simulink model "Controller_Exp"  (R2016a)
settings: Solver=ode4  StartTime=0.0  StopTime=Inf  FixedStep=Ts  RelTol=1e-3
undefined symbols (not defined in the file or in its folder): A_lpf_velocity, B1_lpf_velocity, B2_lpf_velocity, Calibration, commanded_u, GearOffsets, IMUTorsoOffsets, MedullaCommand, ResetDAQ, sample_time, TorsoCOMOffsets, Ts
libraries: xpcethercatlib x188, simulink x37, slrtlib x11, ControllerLibrary x2, dspswit3 x1
(part 2 of 4)

== system Controller_Exp/DAQ/DAQ_sub/Subsystem/EncoderFilters/Filter ==
  note: Look at 10 Samples to determine if there are any spikes in the data.
      | If so, take the median of the 10 samples.
  q : Inport
  Delay : Delay  DelayLength=1
  Delay1 : Delay
  Delay2 : Delay  DelayLength=3
  Delay3 : Delay  DelayLength=4
  Delay4 : Delay  DelayLength=5
  Delay5 : Delay  DelayLength=6
  Delay6 : Delay  DelayLength=7
  Delay7 : Delay  DelayLength=8
  Delay8 : Delay  DelayLength=9
  Median Filter : MATLAB Function  TreatAsAtomicUnit=on
  Vector Concatenate : Concatenate  NumInputs=9  Mode=Multidimensional array  ConcatenateDimension=2
  Velocity Filter : Subsystem
  q_clean : Outport
  dq_clean : Outport  Port=2
  dq_clean_original : Outport  Port=3
  wires:
  Vector Concatenate/1 -> Median Filter/2(q_past)
  Delay/1 -> Vector Concatenate/1
  Delay1/1 -> Vector Concatenate/2
  Delay2/1 -> Vector Concatenate/3
  Delay3/1 -> Vector Concatenate/4
  Delay4/1 -> Vector Concatenate/5
  Delay5/1 -> Vector Concatenate/6
  Delay6/1 -> Vector Concatenate/7
  Delay7/1 -> Vector Concatenate/8
  Delay8/1 -> Vector Concatenate/9
  q/1 -> Delay8/1, Delay7/1, Delay6/1, Delay5/1, Delay4/1, Delay3/1, Delay2/1, Delay1/1, Delay/1, Median Filter/1(q)
  Velocity Filter/2(dq_original) -> dq_clean_original/1
  Velocity Filter/1(dq_out) -> dq_clean/1
  Median Filter/1(q_out) -> Velocity Filter/1(q), q_clean/1

== system Controller_Exp/DAQ/DAQ_sub/Subsystem/EncoderFilters1/CheckAndFilterEncoder ==
  q_daq : Inport
  Logic Filter : MATLAB Function  TreatAsAtomicUnit=on
  Unit Delay1 : UnitDelay  SampleTime=-1
  Unit Delay2 : UnitDelay  SampleTime=-1
  Velocity Filter : Subsystem
  q_clean : Outport
  dq_clean : Outport  Port=2
  dq_clean_origin : Outport  Port=3
  wires:
  Velocity Filter/2(Out2) -> dq_clean_origin/1
  Velocity Filter/1(Out1) -> dq_clean/1
  q_daq/1 -> Unit Delay2/1, Logic Filter/1(q)
  Logic Filter/1(q_out) -> q_clean/1, Velocity Filter/1(In1)
  Logic Filter/2(q_good) -> Unit Delay1/1
  Unit Delay1/1 -> Logic Filter/3(q_good_prev)
  Unit Delay2/1 -> Logic Filter/2(q_prev)

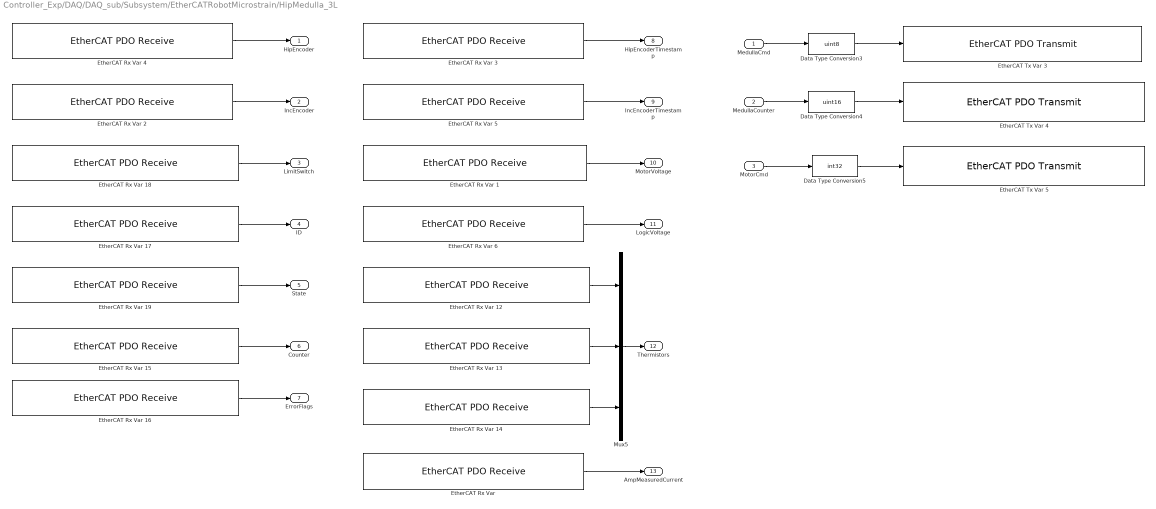
== system Controller_Exp/DAQ/DAQ_sub/Subsystem/EtherCATRobotMicrostrain/HipMedulla_3L ==
  MedullaCmd : Inport
  MedullaCounter : Inport  Port=2
  MotorCmd : Inport  Port=3
  Data Type Conversion3 : DataTypeConversion  OutDataTypeStr=uint8  RndMeth=Simplest
  Data Type Conversion4 : DataTypeConversion  OutDataTypeStr=uint16  RndMeth=Simplest
  Data Type Conversion5 : DataTypeConversion  OutDataTypeStr=int32  RndMeth=Simplest
  "EtherCAT Rx Var " : xpcethercatlib/EtherCAT PDO Receive  Priority=2  sig_name=Box 1 (ATRIAS 2.1 Hip (Medulla 1.5)).Measured Current.Amp Measured Current  sig_offset=760  sig_type=int16  type_size=16  sig_dim=1  device_id=3  sample_time=0.001000
  EtherCAT Rx Var 1 : xpcethercatlib/EtherCAT PDO Receive  Priority=2  sig_name=Box 1 (ATRIAS 2.1 Hip (Medulla 1.5)).Power.Motor Voltage  sig_offset=680  sig_type=uint16  type_size=16  sig_dim=1  device_id=3  sample_time=0.001000
  EtherCAT Rx Var 12 : xpcethercatlib/EtherCAT PDO Receive  Priority=2  sig_name=Box 1 (ATRIAS 2.1 Hip (Medulla 1.5)).Thermistors.Thermistor 0  sig_offset=712  sig_type=uint16  type_size=16  sig_dim=1  device_id=3  sample_time=0.001000
  EtherCAT Rx Var 13 : xpcethercatlib/EtherCAT PDO Receive  Priority=2  sig_name=Box 1 (ATRIAS 2.1 Hip (Medulla 1.5)).Thermistors.Thermistor 1  sig_offset=728  sig_type=uint16  type_size=16  sig_dim=1  device_id=3  sample_time=0.001000
  EtherCAT Rx Var 14 : xpcethercatlib/EtherCAT PDO Receive  Priority=2  sig_name=Box 1 (ATRIAS 2.1 Hip (Medulla 1.5)).Thermistors.Thermistor 2  sig_offset=744  sig_type=uint16  type_size=16  sig_dim=1  device_id=3  sample_time=0.001000
  EtherCAT Rx Var 15 : xpcethercatlib/EtherCAT PDO Receive  Priority=2  sig_name=Box 1 (ATRIAS 2.1 Hip (Medulla 1.5)).uController Status.Counter  sig_offset=608  sig_type=uint8  type_size=8  sig_dim=1  device_id=3  sample_time=0.001000
  EtherCAT Rx Var 16 : xpcethercatlib/EtherCAT PDO Receive  Priority=2  sig_name=Box 1 (ATRIAS 2.1 Hip (Medulla 1.5)).uController Status.Error Flags  sig_offset=616  sig_type=uint8  type_size=8  sig_dim=1  device_id=3  sample_time=0.001000
  EtherCAT Rx Var 17 : xpcethercatlib/EtherCAT PDO Receive  Priority=2  sig_name=Box 1 (ATRIAS 2.1 Hip (Medulla 1.5)).uController Status.ID  sig_offset=592  sig_type=uint8  type_size=8  sig_dim=1  device_id=3  sample_time=0.001000
  EtherCAT Rx Var 18 : xpcethercatlib/EtherCAT PDO Receive  Priority=2  sig_name=Box 1 (ATRIAS 2.1 Hip (Medulla 1.5)).uController Status.Limit Switch  sig_offset=624  sig_type=uint8  type_size=8  sig_dim=1  device_id=3  sample_time=0.001000
  EtherCAT Rx Var 19 : xpcethercatlib/EtherCAT PDO Receive  Priority=2  sig_name=Box 1 (ATRIAS 2.1 Hip (Medulla 1.5)).uController Status.State  sig_offset=600  sig_type=uint8  type_size=8  sig_dim=1  device_id=3  sample_time=0.001000
  EtherCAT Rx Var 2 : xpcethercatlib/EtherCAT PDO Receive  Priority=2  sig_name=Box 1 (ATRIAS 2.1 Hip (Medulla 1.5)).Incremental Encoder.Incremental Encoder  sig_offset=776  sig_type=uint16  type_size=16  sig_dim=1  device_id=3  sample_time=0.001000
  EtherCAT Rx Var 3 : xpcethercatlib/EtherCAT PDO Receive  Priority=2  sig_name=Box 1 (ATRIAS 2.1 Hip (Medulla 1.5)).Hip Encoder.Timestamp  sig_offset=664  sig_type=uint16  type_size=16  sig_dim=1  device_id=3  sample_time=0.001000
  EtherCAT Rx Var 4 : xpcethercatlib/EtherCAT PDO Receive  Priority=2  sig_name=Box 1 (ATRIAS 2.1 Hip (Medulla 1.5)).Hip Encoder.Encoder  sig_offset=632  sig_type=uint32  type_size=32  sig_dim=1  device_id=3  sample_time=0.001000
  EtherCAT Rx Var 5 : xpcethercatlib/EtherCAT PDO Receive  Priority=2  sig_name=Box 1 (ATRIAS 2.1 Hip (Medulla 1.5)).Incremental Encoder.Incremental Encoder Timestamp  sig_offset=792  sig_type=uint16  type_size=16  sig_dim=1  device_id=3  sample_time=0.001000
  EtherCAT Rx Var 6 : xpcethercatlib/EtherCAT PDO Receive  Priority=2  sig_name=Box 1 (ATRIAS 2.1 Hip (Medulla 1.5)).Power.Logic Voltage  sig_offset=696  sig_type=uint16  type_size=16  sig_dim=1  device_id=3  sample_time=0.001000
  EtherCAT Tx Var 3 : xpcethercatlib/EtherCAT PDO Transmit   Priority=3  sig_name=Box 1 (ATRIAS 2.1 Hip (Medulla 1.5)).uControllerInput.Command  sig_offset=592  sig_type=uint8  type_size=8  sig_dim=1  device_id=3  sample_time=0.001000
  EtherCAT Tx Var 4 : xpcethercatlib/EtherCAT PDO Transmit   Priority=3  sig_name=Box 1 (ATRIAS 2.1 Hip (Medulla 1.5)).uControllerInput.Counter  sig_offset=600  sig_type=uint16  type_size=16  sig_dim=1  device_id=3  sample_time=0.001000
  EtherCAT Tx Var 5 : xpcethercatlib/EtherCAT PDO Transmit   Priority=3  sig_name=Box 1 (ATRIAS 2.1 Hip (Medulla 1.5)).uControllerInput.Motor Current  sig_offset=616  sig_type=int32  type_size=32  sig_dim=1  device_id=3  sample_time=0.001000
  Mux5 : Mux  Inputs=3
  HipEncoder : Outport
  IncEncoder : Outport  Port=2
  LimitSwitch : Outport  Port=3
  ID : Outport  Port=4
  State : Outport  Port=5
  Counter : Outport  Port=6
  ErrorFlags : Outport  Port=7
  HipEncoderTimestamp : Outport  Port=8
  IncEncoderTimestamp : Outport  Port=9
  MotorVoltage : Outport  Port=10
  LogicVoltage : Outport  Port=11
  Thermistors : Outport  Port=12
  AmpMeasuredCurrent : Outport  Port=13
  wires:
  Mux5/1 -> Thermistors/1
  "EtherCAT Rx Var "/1 -> AmpMeasuredCurrent/1
  EtherCAT Rx Var 14/1 -> Mux5/3
  EtherCAT Rx Var 13/1 -> Mux5/2
  EtherCAT Rx Var 12/1 -> Mux5/1
  EtherCAT Rx Var 1/1 -> MotorVoltage/1
  EtherCAT Rx Var 6/1 -> LogicVoltage/1
  EtherCAT Rx Var 16/1 -> ErrorFlags/1
  EtherCAT Rx Var 19/1 -> State/1
  EtherCAT Rx Var 18/1 -> LimitSwitch/1
  EtherCAT Rx Var 17/1 -> ID/1
  EtherCAT Rx Var 15/1 -> Counter/1
  EtherCAT Rx Var 2/1 -> IncEncoder/1
  EtherCAT Rx Var 3/1 -> HipEncoderTimestamp/1
  EtherCAT Rx Var 4/1 -> HipEncoder/1
  EtherCAT Rx Var 5/1 -> IncEncoderTimestamp/1
  MotorCmd/1 -> Data Type Conversion5/1
  MedullaCounter/1 -> Data Type Conversion4/1
  MedullaCmd/1 -> Data Type Conversion3/1
  Data Type Conversion5/1 -> EtherCAT Tx Var 5/1
  Data Type Conversion4/1 -> EtherCAT Tx Var 4/1
  Data Type Conversion3/1 -> EtherCAT Tx Var 3/1

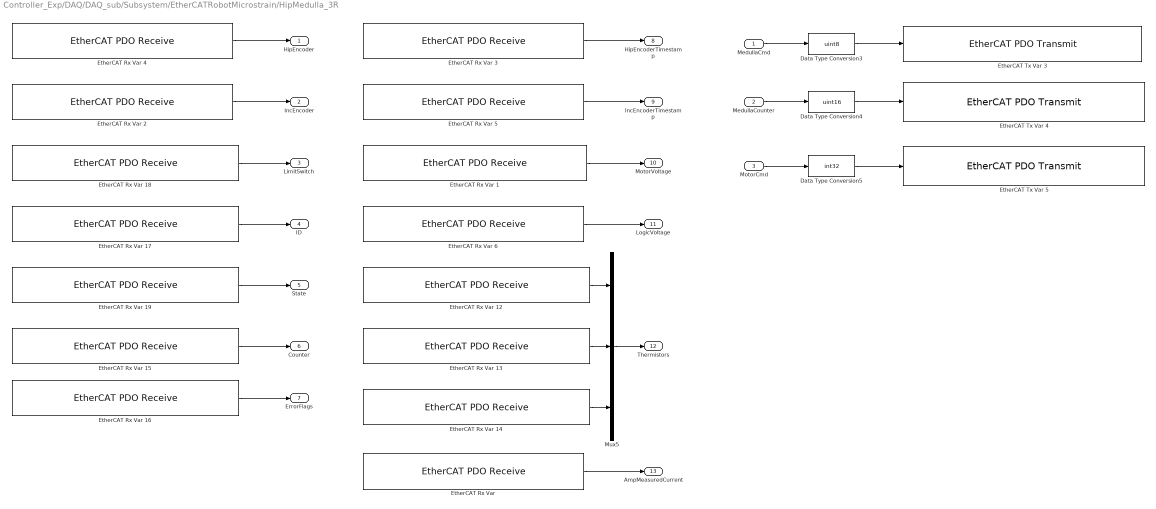
== system Controller_Exp/DAQ/DAQ_sub/Subsystem/EtherCATRobotMicrostrain/HipMedulla_3R ==
  MedullaCmd : Inport
  MedullaCounter : Inport  Port=2
  MotorCmd : Inport  Port=3
  Data Type Conversion3 : DataTypeConversion  OutDataTypeStr=uint8  RndMeth=Simplest
  Data Type Conversion4 : DataTypeConversion  OutDataTypeStr=uint16  RndMeth=Simplest
  Data Type Conversion5 : DataTypeConversion  OutDataTypeStr=int32  RndMeth=Simplest
  "EtherCAT Rx Var " : xpcethercatlib/EtherCAT PDO Receive  Priority=2  sig_name=Box 11 (ATRIAS 2.1 Hip (Medulla 1.5)).Measured Current.Amp Measured Current  sig_offset=2768  sig_type=int16  type_size=16  sig_dim=1  device_id=3  sample_time=0.001000
  EtherCAT Rx Var 1 : xpcethercatlib/EtherCAT PDO Receive  Priority=2  sig_name=Box 11 (ATRIAS 2.1 Hip (Medulla 1.5)).Power.Motor Voltage  sig_offset=2688  sig_type=uint16  type_size=16  sig_dim=1  device_id=3  sample_time=0.001000
  EtherCAT Rx Var 12 : xpcethercatlib/EtherCAT PDO Receive  Priority=2  sig_name=Box 11 (ATRIAS 2.1 Hip (Medulla 1.5)).Thermistors.Thermistor 0  sig_offset=2720  sig_type=uint16  type_size=16  sig_dim=1  device_id=3  sample_time=0.001000
  EtherCAT Rx Var 13 : xpcethercatlib/EtherCAT PDO Receive  Priority=2  sig_name=Box 11 (ATRIAS 2.1 Hip (Medulla 1.5)).Thermistors.Thermistor 1  sig_offset=2736  sig_type=uint16  type_size=16  sig_dim=1  device_id=3  sample_time=0.001000
  EtherCAT Rx Var 14 : xpcethercatlib/EtherCAT PDO Receive  Priority=2  sig_name=Box 11 (ATRIAS 2.1 Hip (Medulla 1.5)).Thermistors.Thermistor 2  sig_offset=2752  sig_type=uint16  type_size=16  sig_dim=1  device_id=3  sample_time=0.001000
  EtherCAT Rx Var 15 : xpcethercatlib/EtherCAT PDO Receive  Priority=2  sig_name=Box 11 (ATRIAS 2.1 Hip (Medulla 1.5)).uController Status.Counter  sig_offset=2616  sig_type=uint8  type_size=8  sig_dim=1  device_id=3  sample_time=0.001000
  EtherCAT Rx Var 16 : xpcethercatlib/EtherCAT PDO Receive  Priority=2  sig_name=Box 11 (ATRIAS 2.1 Hip (Medulla 1.5)).uController Status.Error Flags  sig_offset=2624  sig_type=uint8  type_size=8  sig_dim=1  device_id=3  sample_time=0.001000
  EtherCAT Rx Var 17 : xpcethercatlib/EtherCAT PDO Receive  Priority=2  sig_name=Box 11 (ATRIAS 2.1 Hip (Medulla 1.5)).uController Status.ID  sig_offset=2600  sig_type=uint8  type_size=8  sig_dim=1  device_id=3  sample_time=0.001000
  EtherCAT Rx Var 18 : xpcethercatlib/EtherCAT PDO Receive  Priority=2  sig_name=Box 11 (ATRIAS 2.1 Hip (Medulla 1.5)).uController Status.Limit Switch  sig_offset=2632  sig_type=uint8  type_size=8  sig_dim=1  device_id=3  sample_time=0.001000
  EtherCAT Rx Var 19 : xpcethercatlib/EtherCAT PDO Receive  Priority=2  sig_name=Box 11 (ATRIAS 2.1 Hip (Medulla 1.5)).uController Status.State  sig_offset=2608  sig_type=uint8  type_size=8  sig_dim=1  device_id=3  sample_time=0.001000
  EtherCAT Rx Var 2 : xpcethercatlib/EtherCAT PDO Receive  Priority=2  sig_name=Box 11 (ATRIAS 2.1 Hip (Medulla 1.5)).Incremental Encoder.Incremental Encoder  sig_offset=2784  sig_type=uint16  type_size=16  sig_dim=1  device_id=3  sample_time=0.001000
  EtherCAT Rx Var 3 : xpcethercatlib/EtherCAT PDO Receive  Priority=2  sig_name=Box 11 (ATRIAS 2.1 Hip (Medulla 1.5)).Hip Encoder.Timestamp  sig_offset=2672  sig_type=uint16  type_size=16  sig_dim=1  device_id=3  sample_time=0.001000
  EtherCAT Rx Var 4 : xpcethercatlib/EtherCAT PDO Receive  Priority=2  sig_name=Box 11 (ATRIAS 2.1 Hip (Medulla 1.5)).Hip Encoder.Encoder  sig_offset=2640  sig_type=uint32  type_size=32  sig_dim=1  device_id=3  sample_time=0.001000
  EtherCAT Rx Var 5 : xpcethercatlib/EtherCAT PDO Receive  Priority=2  sig_name=Box 11 (ATRIAS 2.1 Hip (Medulla 1.5)).Incremental Encoder.Incremental Encoder Timestamp  sig_offset=2800  sig_type=uint16  type_size=16  sig_dim=1  device_id=3  sample_time=0.001000
  EtherCAT Rx Var 6 : xpcethercatlib/EtherCAT PDO Receive  Priority=2  sig_name=Box 11 (ATRIAS 2.1 Hip (Medulla 1.5)).Power.Logic Voltage  sig_offset=2704  sig_type=uint16  type_size=16  sig_dim=1  device_id=3  sample_time=0.001000
  EtherCAT Tx Var 3 : xpcethercatlib/EtherCAT PDO Transmit   Priority=3  sig_name=Box 11 (ATRIAS 2.1 Hip (Medulla 1.5)).uControllerInput.Command  sig_offset=2600  sig_type=uint8  type_size=8  sig_dim=1  device_id=3  sample_time=0.001000
  EtherCAT Tx Var 4 : xpcethercatlib/EtherCAT PDO Transmit   Priority=3  sig_name=Box 11 (ATRIAS 2.1 Hip (Medulla 1.5)).uControllerInput.Counter  sig_offset=2608  sig_type=uint16  type_size=16  sig_dim=1  device_id=3  sample_time=0.001000
  EtherCAT Tx Var 5 : xpcethercatlib/EtherCAT PDO Transmit   Priority=3  sig_name=Box 11 (ATRIAS 2.1 Hip (Medulla 1.5)).uControllerInput.Motor Current  sig_offset=2624  sig_type=int32  type_size=32  sig_dim=1  device_id=3  sample_time=0.001000
  Mux5 : Mux  Inputs=3
  HipEncoder : Outport
  IncEncoder : Outport  Port=2
  LimitSwitch : Outport  Port=3
  ID : Outport  Port=4
  State : Outport  Port=5
  Counter : Outport  Port=6
  ErrorFlags : Outport  Port=7
  HipEncoderTimestamp : Outport  Port=8
  IncEncoderTimestamp : Outport  Port=9
  MotorVoltage : Outport  Port=10
  LogicVoltage : Outport  Port=11
  Thermistors : Outport  Port=12
  AmpMeasuredCurrent : Outport  Port=13
  wires:
  Mux5/1 -> Thermistors/1
  "EtherCAT Rx Var "/1 -> AmpMeasuredCurrent/1
  EtherCAT Rx Var 14/1 -> Mux5/3
  EtherCAT Rx Var 13/1 -> Mux5/2
  EtherCAT Rx Var 12/1 -> Mux5/1
  EtherCAT Rx Var 1/1 -> MotorVoltage/1
  EtherCAT Rx Var 6/1 -> LogicVoltage/1
  EtherCAT Rx Var 16/1 -> ErrorFlags/1
  EtherCAT Rx Var 19/1 -> State/1
  EtherCAT Rx Var 18/1 -> LimitSwitch/1
  EtherCAT Rx Var 17/1 -> ID/1
  EtherCAT Rx Var 15/1 -> Counter/1
  EtherCAT Rx Var 2/1 -> IncEncoder/1
  EtherCAT Rx Var 3/1 -> HipEncoderTimestamp/1
  EtherCAT Rx Var 4/1 -> HipEncoder/1
  EtherCAT Rx Var 5/1 -> IncEncoderTimestamp/1
  MotorCmd/1 -> Data Type Conversion5/1
  MedullaCounter/1 -> Data Type Conversion4/1
  MedullaCmd/1 -> Data Type Conversion3/1
  Data Type Conversion5/1 -> EtherCAT Tx Var 5/1
  Data Type Conversion4/1 -> EtherCAT Tx Var 4/1
  Data Type Conversion3/1 -> EtherCAT Tx Var 3/1

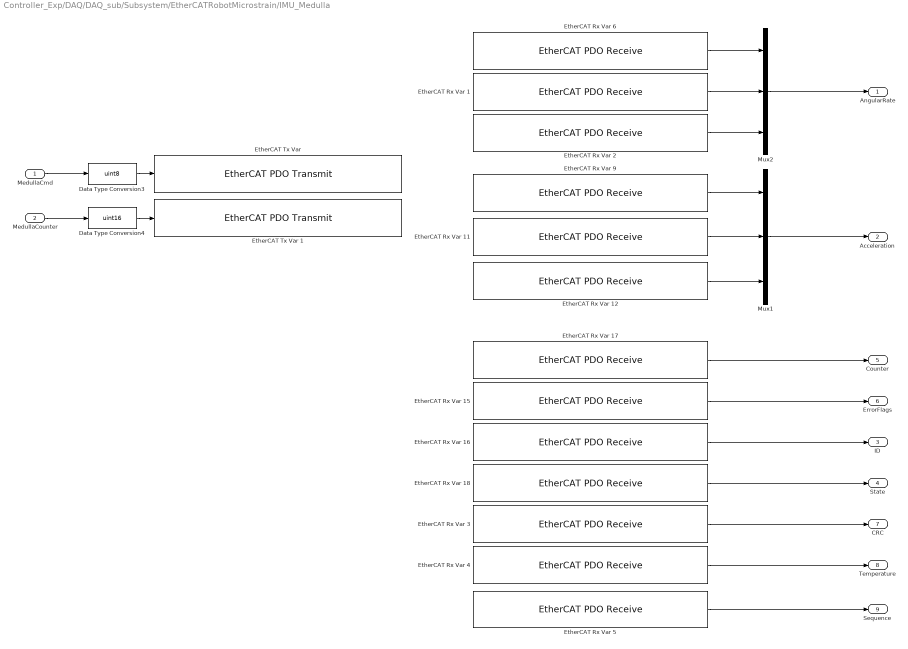
== system Controller_Exp/DAQ/DAQ_sub/Subsystem/EtherCATRobotMicrostrain/IMU_Medulla ==
  MedullaCmd : Inport
  MedullaCounter : Inport  Port=2
  Data Type Conversion3 : DataTypeConversion  OutDataTypeStr=uint8  RndMeth=Simplest
  Data Type Conversion4 : DataTypeConversion  OutDataTypeStr=uint16  RndMeth=Simplest
  EtherCAT Rx Var 1 : xpcethercatlib/EtherCAT PDO Receive  Priority=2  sig_name=Box 4 (ATRIAS 2.1 IMU (Medulla 1.5)).Rotation.Y  sig_offset=872  sig_type=single  type_size=32  sig_dim=1  device_id=3  sample_time=0.001000
  EtherCAT Rx Var 11 : xpcethercatlib/EtherCAT PDO Receive  Priority=2  sig_name=Box 4 (ATRIAS 2.1 IMU (Medulla 1.5)).Acceleration.Y  sig_offset=968  sig_type=single  type_size=32  sig_dim=1  device_id=3  sample_time=0.001000
  EtherCAT Rx Var 12 : xpcethercatlib/EtherCAT PDO Receive  Priority=2  sig_name=Box 4 (ATRIAS 2.1 IMU (Medulla 1.5)).Acceleration.Z  sig_offset=1000  sig_type=single  type_size=32  sig_dim=1  device_id=3  sample_time=0.001000
  EtherCAT Rx Var 15 : xpcethercatlib/EtherCAT PDO Receive  Priority=2  sig_name=Box 4 (ATRIAS 2.1 IMU (Medulla 1.5)).uController Status.Error Flags  sig_offset=832  sig_type=uint8  type_size=8  sig_dim=1  device_id=3  sample_time=0.001000
  EtherCAT Rx Var 16 : xpcethercatlib/EtherCAT PDO Receive  Priority=2  sig_name=Box 4 (ATRIAS 2.1 IMU (Medulla 1.5)).uController Status.ID  sig_offset=808  sig_type=uint8  type_size=8  sig_dim=1  device_id=3  sample_time=0.001000
  EtherCAT Rx Var 17 : xpcethercatlib/EtherCAT PDO Receive  Priority=2  sig_name=Box 4 (ATRIAS 2.1 IMU (Medulla 1.5)).uController Status.Counter  sig_offset=824  sig_type=uint8  type_size=8  sig_dim=1  device_id=3  sample_time=0.001000
  EtherCAT Rx Var 18 : xpcethercatlib/EtherCAT PDO Receive  Priority=2  sig_name=Box 4 (ATRIAS 2.1 IMU (Medulla 1.5)).Status.Status  sig_offset=1032  sig_type=uint8  type_size=8  sig_dim=1  device_id=3  sample_time=0.001000
  EtherCAT Rx Var 2 : xpcethercatlib/EtherCAT PDO Receive  Priority=2  sig_name=Box 4 (ATRIAS 2.1 IMU (Medulla 1.5)).Rotation.Z  sig_offset=904  sig_type=single  type_size=32  sig_dim=1  device_id=3  sample_time=0.001000
  EtherCAT Rx Var 3 : xpcethercatlib/EtherCAT PDO Receive  Priority=2  sig_name=Box 4 (ATRIAS 2.1 IMU (Medulla 1.5)).Status.Status  sig_offset=1032  sig_type=uint8  type_size=8  sig_dim=1  device_id=3  sample_time=0.001000
  EtherCAT Rx Var 4 : xpcethercatlib/EtherCAT PDO Receive  Priority=2  sig_name=Box 4 (ATRIAS 2.1 IMU (Medulla 1.5)).Status.Temperature  sig_offset=1048  sig_type=int16  type_size=16  sig_dim=1  device_id=3  sample_time=0.001000
  EtherCAT Rx Var 5 : xpcethercatlib/EtherCAT PDO Receive  Priority=2  sig_name=Box 4 (ATRIAS 2.1 IMU (Medulla 1.5)).Status.Sequence  sig_offset=1040  sig_type=uint8  type_size=8  sig_dim=1  device_id=3  sample_time=0.001000
  EtherCAT Rx Var 6 : xpcethercatlib/EtherCAT PDO Receive  Priority=2  sig_name=Box 4 (ATRIAS 2.1 IMU (Medulla 1.5)).Rotation.X  sig_offset=840  sig_type=single  type_size=32  sig_dim=1  device_id=3  sample_time=0.001000
  EtherCAT Rx Var 9 : xpcethercatlib/EtherCAT PDO Receive  Priority=2  sig_name=Box 4 (ATRIAS 2.1 IMU (Medulla 1.5)).Acceleration.X  sig_offset=936  sig_type=single  type_size=32  sig_dim=1  device_id=3  sample_time=0.001000
  "EtherCAT Tx Var " : xpcethercatlib/EtherCAT PDO Transmit   Priority=3  sig_name=Box 4 (ATRIAS 2.1 IMU (Medulla 1.5)).uControllerInput.Command  sig_offset=808  sig_type=uint8  type_size=8  sig_dim=1  device_id=3  sample_time=0.001000
  EtherCAT Tx Var 1 : xpcethercatlib/EtherCAT PDO Transmit   Priority=3  sig_name=Box 4 (ATRIAS 2.1 IMU (Medulla 1.5)).uControllerInput.Counter  sig_offset=816  sig_type=uint16  type_size=16  sig_dim=1  device_id=3  sample_time=0.001000
  Mux1 : Mux  Inputs=3
  Mux2 : Mux  Inputs=3
  AngularRate : Outport
  Acceleration : Outport  Port=2
  ID : Outport  Port=3
  State : Outport  Port=4
  Counter : Outport  Port=5
  ErrorFlags : Outport  Port=6
  CRC : Outport  Port=7
  Temperature : Outport  Port=8
  Sequence : Outport  Port=9
  wires:
  EtherCAT Rx Var 6/1 -> Mux2/1
  EtherCAT Rx Var 2/1 -> Mux2/3
  EtherCAT Rx Var 1/1 -> Mux2/2
  Mux2/1 -> AngularRate/1
  EtherCAT Rx Var 9/1 -> Mux1/1
  EtherCAT Rx Var 11/1 -> Mux1/2
  EtherCAT Rx Var 12/1 -> Mux1/3
  EtherCAT Rx Var 18/1 -> State/1
  EtherCAT Rx Var 16/1 -> ID/1
  EtherCAT Rx Var 15/1 -> ErrorFlags/1
  EtherCAT Rx Var 17/1 -> Counter/1
  MedullaCounter/1 -> Data Type Conversion4/1
  MedullaCmd/1 -> Data Type Conversion3/1
  Data Type Conversion4/1 -> EtherCAT Tx Var 1/1
  Data Type Conversion3/1 -> "EtherCAT Tx Var "/1
  Mux1/1 -> Acceleration/1
  EtherCAT Rx Var 3/1 -> CRC/1
  EtherCAT Rx Var 4/1 -> Temperature/1
  EtherCAT Rx Var 5/1 -> Sequence/1

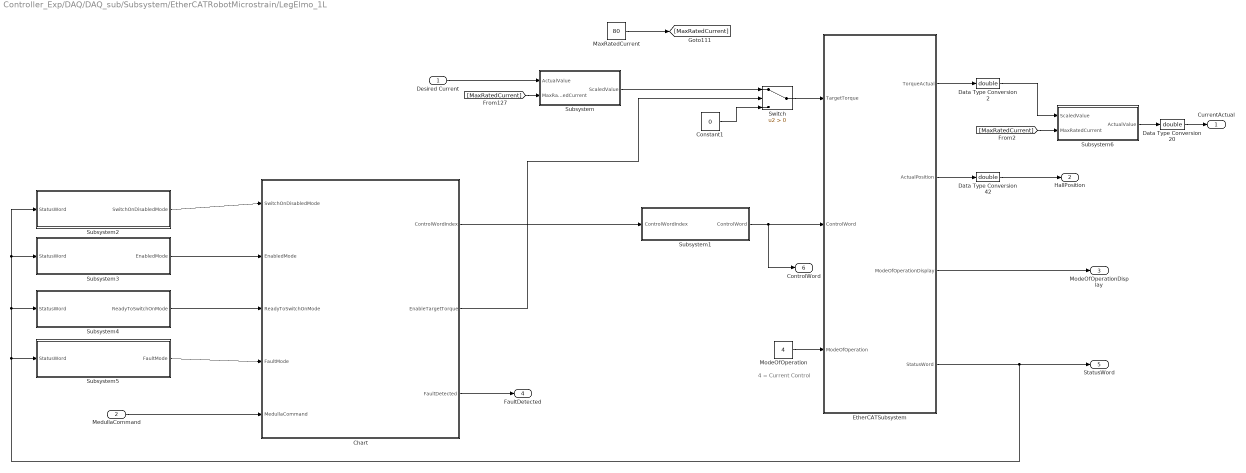
== system Controller_Exp/DAQ/DAQ_sub/Subsystem/EtherCATRobotMicrostrain/LegElmo_1L ==
  note: 4 = Current Control
  Desired Current : Inport
  MedullaCommand : Inport  Port=2
  Chart : Stateflow chart  TreatAsAtomicUnit=on
  Constant1 : Constant  Value=0  OutDataTypeStr=int16
  Data Type Conversion2 : DataTypeConversion  OutDataTypeStr=double
  Data Type Conversion20 : DataTypeConversion  OutDataTypeStr=double
  Data Type Conversion42 : DataTypeConversion  OutDataTypeStr=double
  EtherCATSubsystem : Subsystem
  MaxRatedCurrent : Constant  Value=80  OutDataTypeStr=double
  ModeOfOperation : Constant  Value=4  OutDataTypeStr=int8
  Subsystem : Subsystem
  Subsystem1 : Subsystem
  Subsystem2 : Subsystem
  Subsystem3 : Subsystem
  Subsystem4 : Subsystem
  Subsystem5 : Subsystem
  Subsystem6 : Subsystem
  Switch : Switch  Criteria=u2 > Threshold
  CurrentActual : Outport
  HallPosition : Outport  Port=2
  ModeOfOperationDisplay : Outport  Port=3
  FaultDetected : Outport  Port=4
  StatusWord : Outport  Port=5
  ControlWord : Outport  Port=6
  wires:
  Data Type Conversion2/1 -> Subsystem6/1(ScaledValue)
  EtherCATSubsystem/1(TorqueActual) -> Data Type Conversion2/1
  MedullaCommand/1 -> Chart/5(MedullaCommand)
  Chart/3(FaultDetected) -> FaultDetected/1
  [MaxRatedCurrent] -> Subsystem/2(MaxRatedCurrent)
  MaxRatedCurrent/1 -> [MaxRatedCurrent]
  Subsystem6/1(ActualValue) -> Data Type Conversion20/1
  [MaxRatedCurrent] -> Subsystem6/2(MaxRatedCurrent)
  Switch/1 -> EtherCATSubsystem/1(TargetTorque)
  Subsystem5/1(FaultMode) -> Chart/4(FaultMode)
  Subsystem4/1(ReadyToSwitchOnMode) -> Chart/3(ReadyToSwitchOnMode)
  Subsystem3/1(EnabledMode) -> Chart/2(EnabledMode)
  Subsystem2/1(SwitchOnDisabledMode) -> Chart/1(SwitchOnDisabledMode)
  Chart/1(ControlWordIndex) -> Subsystem1/1(ControlWordIndex)
  Chart/2(EnableTargetTorque) -> Switch/2
  Constant1/1 -> Switch/3
  Subsystem/1(ScaledValue) -> Switch/1
  EtherCATSubsystem/2(ActualPosition) -> Data Type Conversion42/1
  ModeOfOperation/1 -> EtherCATSubsystem/3(ModeOfOperation)
  EtherCATSubsystem/3(ModeOfOperationDisplay) -> ModeOfOperationDisplay/1
  Data Type Conversion42/1 -> HallPosition/1
  Data Type Conversion20/1 -> CurrentActual/1
  Desired Current/1 -> Subsystem/1(ActualValue)
  EtherCATSubsystem/4(StatusWord) -> StatusWord/1, Subsystem2/1(StatusWord), Subsystem3/1(StatusWord), Subsystem4/1(StatusWord), Subsystem5/1(StatusWord)
  Subsystem1/1(ControlWord) -> ControlWord/1, EtherCATSubsystem/2(ControlWord)

== system Controller_Exp/DAQ/DAQ_sub/Subsystem/EtherCATRobotMicrostrain/LegElmo_1R ==
  note: 4 = Current Control
  Desired Current : Inport
  MedullaCommand : Inport  Port=2
  Chart : Stateflow chart  TreatAsAtomicUnit=on
  Constant1 : Constant  Value=0  OutDataTypeStr=int16
  Data Type Conversion20 : DataTypeConversion  OutDataTypeStr=double
  Data Type Conversion3 : DataTypeConversion  OutDataTypeStr=double
  Data Type Conversion42 : DataTypeConversion  OutDataTypeStr=double
  EtherCATSubsystem : Subsystem
  MaxRatedCurrent : Constant  Value=80  OutDataTypeStr=double
  ModeOfOperation : Constant  Value=4  OutDataTypeStr=int8
  Subsystem : Subsystem
  Subsystem1 : Subsystem
  Subsystem2 : Subsystem
  Subsystem3 : Subsystem
  Subsystem4 : Subsystem
  Subsystem5 : Subsystem
  Subsystem6 : Subsystem
  Switch : Switch  Criteria=u2 > Threshold
  CurrentActual : Outport
  HallPosition : Outport  Port=2
  ModeOfOperationDisplay : Outport  Port=3
  FaultDetected : Outport  Port=4
  StatusWord : Outport  Port=5
  ControlWord : Outport  Port=6
  wires:
  Data Type Conversion3/1 -> Subsystem6/1(ScaledValue)
  EtherCATSubsystem/1(TorqueActual) -> Data Type Conversion3/1
  MedullaCommand/1 -> Chart/5(MedullaCommand)
  Chart/3(FaultDetected) -> FaultDetected/1
  [MaxRatedCurrent] -> Subsystem/2(MaxRatedCurrent)
  MaxRatedCurrent/1 -> [MaxRatedCurrent]
  Subsystem6/1(ActualValue) -> Data Type Conversion20/1
  [MaxRatedCurrent] -> Subsystem6/2(MaxRatedCurrent)
  Switch/1 -> EtherCATSubsystem/1(TargetTorque)
  Subsystem5/1(FaultMode) -> Chart/4(FaultMode)
  Subsystem4/1(ReadyToSwitchOnMode) -> Chart/3(ReadyToSwitchOnMode)
  Subsystem3/1(EnabledMode) -> Chart/2(EnabledMode)
  Subsystem2/1(SwitchOnDisabledMode) -> Chart/1(SwitchOnDisabledMode)
  Chart/1(ControlWordIndex) -> Subsystem1/1(ControlWordIndex)
  Chart/2(EnableTargetTorque) -> Switch/2
  Constant1/1 -> Switch/3
  Subsystem/1(ScaledValue) -> Switch/1
  EtherCATSubsystem/2(ActualPosition) -> Data Type Conversion42/1
  ModeOfOperation/1 -> EtherCATSubsystem/3(ModeOfOperation)
  Data Type Conversion42/1 -> HallPosition/1
  Data Type Conversion20/1 -> CurrentActual/1
  Desired Current/1 -> Subsystem/1(ActualValue)
  EtherCATSubsystem/3(ModeOfOperationDisplay) -> ModeOfOperationDisplay/1
  EtherCATSubsystem/4(StatusWord) -> StatusWord/1, Subsystem2/1(StatusWord), Subsystem3/1(StatusWord), Subsystem4/1(StatusWord), Subsystem5/1(StatusWord)
  Subsystem1/1(ControlWord) -> ControlWord/1, EtherCATSubsystem/2(ControlWord)

== system Controller_Exp/DAQ/DAQ_sub/Subsystem/EtherCATRobotMicrostrain/LegElmo_2L ==
  note: 4 = Current Control
  Desired Current : Inport
  MedullaCommand : Inport  Port=2
  Chart : Stateflow chart  TreatAsAtomicUnit=on
  Constant1 : Constant  Value=0  OutDataTypeStr=int16
  Data Type Conversion2 : DataTypeConversion  OutDataTypeStr=double
  Data Type Conversion20 : DataTypeConversion  OutDataTypeStr=double
  Data Type Conversion42 : DataTypeConversion  OutDataTypeStr=double
  EtherCATSubsystem : Subsystem
  MaxRatedCurrent : Constant  Value=80  OutDataTypeStr=double
  ModeOfOperation : Constant  Value=4  OutDataTypeStr=int8
  Subsystem : Subsystem
  Subsystem1 : Subsystem
  Subsystem2 : Subsystem
  Subsystem3 : Subsystem
  Subsystem4 : Subsystem
  Subsystem5 : Subsystem
  Subsystem6 : Subsystem
  Switch : Switch  Criteria=u2 > Threshold
  CurrentActual : Outport
  ElmoPosition : Outport  Port=2
  ModeOfOperationDisplay : Outport  Port=3
  FaultDetected : Outport  Port=4
  StatusWord : Outport  Port=5
  ControlWord : Outport  Port=6
  wires:
  Data Type Conversion2/1 -> Subsystem6/1(ScaledValue)
  EtherCATSubsystem/1(TorqueActual) -> Data Type Conversion2/1
  MedullaCommand/1 -> Chart/5(MedullaCommand)
  Chart/3(FaultDetected) -> FaultDetected/1
  [MaxRatedCurrent] -> Subsystem/2(MaxRatedCurrent)
  MaxRatedCurrent/1 -> [MaxRatedCurrent]
  Subsystem6/1(ActualValue) -> Data Type Conversion20/1
  [MaxRatedCurrent] -> Subsystem6/2(MaxRatedCurrent)
  Switch/1 -> EtherCATSubsystem/1(TargetTorque)
  Subsystem5/1(FaultMode) -> Chart/4(FaultMode)
  Subsystem4/1(ReadyToSwitchOnMode) -> Chart/3(ReadyToSwitchOnMode)
  Subsystem3/1(EnabledMode) -> Chart/2(EnabledMode)
  Subsystem2/1(SwitchOnDisabledMode) -> Chart/1(SwitchOnDisabledMode)
  Chart/1(ControlWordIndex) -> Subsystem1/1(ControlWordIndex)
  Chart/2(EnableTargetTorque) -> Switch/2
  Constant1/1 -> Switch/3
  Subsystem/1(ScaledValue) -> Switch/1
  EtherCATSubsystem/2(ActualPosition) -> Data Type Conversion42/1
  ModeOfOperation/1 -> EtherCATSubsystem/3(ModeOfOperation)
  EtherCATSubsystem/3(ModeOfOperationDisplay) -> ModeOfOperationDisplay/1
  Data Type Conversion42/1 -> ElmoPosition/1
  Data Type Conversion20/1 -> CurrentActual/1
  Desired Current/1 -> Subsystem/1(ActualValue)
  EtherCATSubsystem/4(StatusWord) -> StatusWord/1, Subsystem2/1(StatusWord), Subsystem3/1(StatusWord), Subsystem4/1(StatusWord), Subsystem5/1(StatusWord)
  Subsystem1/1(ControlWord) -> ControlWord/1, EtherCATSubsystem/2(ControlWord)

== system Controller_Exp/DAQ/DAQ_sub/Subsystem/EtherCATRobotMicrostrain/LegElmo_2R ==
  note: 4 = Current Control
  Desired Current : Inport
  MedullaCommand : Inport  Port=2
  Chart : Stateflow chart  TreatAsAtomicUnit=on
  Constant1 : Constant  Value=0  OutDataTypeStr=int16
  Data Type Conversion2 : DataTypeConversion  OutDataTypeStr=double
  Data Type Conversion20 : DataTypeConversion  OutDataTypeStr=double
  Data Type Conversion42 : DataTypeConversion  OutDataTypeStr=double
  EtherCATSubsystem : Subsystem
  MaxRatedCurrent : Constant  Value=80  OutDataTypeStr=double
  ModeOfOperation : Constant  Value=4  OutDataTypeStr=int8
  Subsystem : Subsystem
  Subsystem1 : Subsystem
  Subsystem2 : Subsystem
  Subsystem3 : Subsystem
  Subsystem4 : Subsystem
  Subsystem5 : Subsystem
  Subsystem6 : Subsystem
  Switch : Switch  Criteria=u2 > Threshold
  CurrentActual : Outport
  HallPosition : Outport  Port=2
  ModeOfOperationDisplay : Outport  Port=3
  FaultDetected : Outport  Port=4
  StatusWord : Outport  Port=5
  ControlWord : Outport  Port=6
  wires:
  Data Type Conversion2/1 -> Subsystem6/1(ScaledValue)
  EtherCATSubsystem/1(TorqueActual) -> Data Type Conversion2/1
  MedullaCommand/1 -> Chart/5(MedullaCommand)
  Chart/3(FaultDetected) -> FaultDetected/1
  [MaxRatedCurrent] -> Subsystem/2(MaxRatedCurrent)
  MaxRatedCurrent/1 -> [MaxRatedCurrent]
  Subsystem6/1(ActualValue) -> Data Type Conversion20/1
  [MaxRatedCurrent] -> Subsystem6/2(MaxRatedCurrent)
  Switch/1 -> EtherCATSubsystem/1(TargetTorque)
  Subsystem5/1(FaultMode) -> Chart/4(FaultMode)
  Subsystem4/1(ReadyToSwitchOnMode) -> Chart/3(ReadyToSwitchOnMode)
  Subsystem3/1(EnabledMode) -> Chart/2(EnabledMode)
  Subsystem2/1(SwitchOnDisabledMode) -> Chart/1(SwitchOnDisabledMode)
  Chart/1(ControlWordIndex) -> Subsystem1/1(ControlWordIndex)
  Chart/2(EnableTargetTorque) -> Switch/2
  Constant1/1 -> Switch/3
  Subsystem/1(ScaledValue) -> Switch/1
  EtherCATSubsystem/2(ActualPosition) -> Data Type Conversion42/1
  ModeOfOperation/1 -> EtherCATSubsystem/3(ModeOfOperation)
  Data Type Conversion42/1 -> HallPosition/1
  Data Type Conversion20/1 -> CurrentActual/1
  Desired Current/1 -> Subsystem/1(ActualValue)
  EtherCATSubsystem/3(ModeOfOperationDisplay) -> ModeOfOperationDisplay/1
  EtherCATSubsystem/4(StatusWord) -> StatusWord/1, Subsystem2/1(StatusWord), Subsystem3/1(StatusWord), Subsystem4/1(StatusWord), Subsystem5/1(StatusWord)
  Subsystem1/1(ControlWord) -> ControlWord/1, EtherCATSubsystem/2(ControlWord)

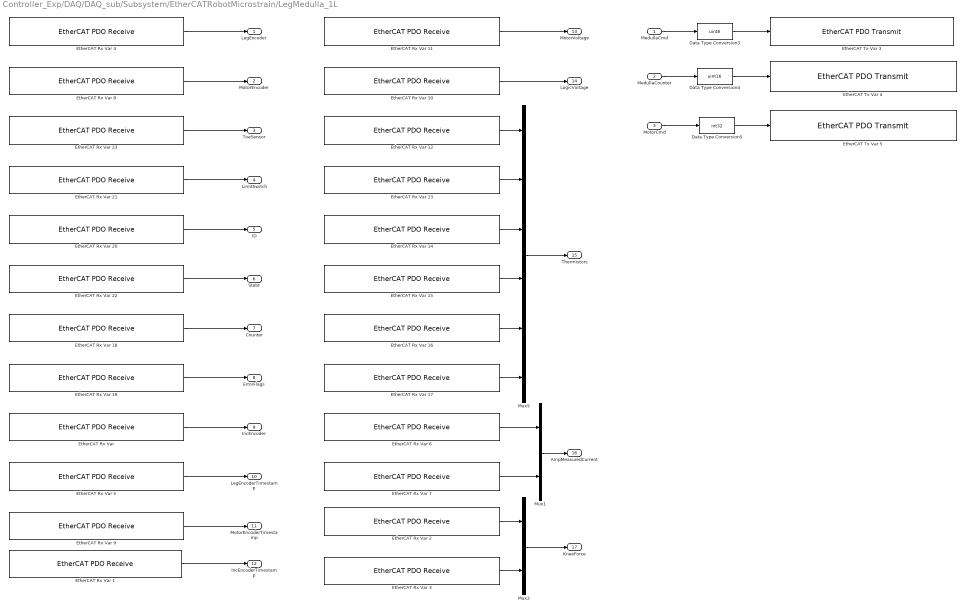
== system Controller_Exp/DAQ/DAQ_sub/Subsystem/EtherCATRobotMicrostrain/LegMedulla_1L ==
  MedullaCmd : Inport
  MedullaCounter : Inport  Port=2
  MotorCmd : Inport  Port=3
  Data Type Conversion3 : DataTypeConversion  OutDataTypeStr=uint8  RndMeth=Simplest
  Data Type Conversion4 : DataTypeConversion  OutDataTypeStr=uint16  RndMeth=Simplest
  Data Type Conversion5 : DataTypeConversion  OutDataTypeStr=int32  RndMeth=Simplest
  "EtherCAT Rx Var " : xpcethercatlib/EtherCAT PDO Receive  Priority=2  sig_name=Box 5 (ATRIAS 2.1 Leg (Medulla 1.5)).Incremental Encoder.Incremental Encoder  sig_offset=1248  sig_type=uint16  type_size=16  sig_dim=1  device_id=3  sample_time=0.001000
  EtherCAT Rx Var 1 : xpcethercatlib/EtherCAT PDO Receive  Priority=2  sig_name=Box 5 (ATRIAS 2.1 Leg (Medulla 1.5)).Incremental Encoder.Incremental Encoder Timestamp  sig_offset=1264  sig_type=uint16  type_size=16  sig_dim=1  device_id=3  sample_time=0.001000
  EtherCAT Rx Var 10 : xpcethercatlib/EtherCAT PDO Receive  Priority=2  sig_name=Box 5 (ATRIAS 2.1 Leg (Medulla 1.5)).Power.Logic Voltage  sig_offset=1296  sig_type=uint16  type_size=16  sig_dim=1  device_id=3  sample_time=0.001000
  EtherCAT Rx Var 11 : xpcethercatlib/EtherCAT PDO Receive  Priority=2  sig_name=Box 5 (ATRIAS 2.1 Leg (Medulla 1.5)).Power.Motor Voltage  sig_offset=1280  sig_type=uint16  type_size=16  sig_dim=1  device_id=3  sample_time=0.001000
  EtherCAT Rx Var 12 : xpcethercatlib/EtherCAT PDO Receive  Priority=2  sig_name=Box 5 (ATRIAS 2.1 Leg (Medulla 1.5)).Thermistors.Thermistor 0  sig_offset=1312  sig_type=uint16  type_size=16  sig_dim=1  device_id=3  sample_time=0.001000
  EtherCAT Rx Var 13 : xpcethercatlib/EtherCAT PDO Receive  Priority=2  sig_name=Box 5 (ATRIAS 2.1 Leg (Medulla 1.5)).Thermistors.Thermistor 1  sig_offset=1328  sig_type=uint16  type_size=16  sig_dim=1  device_id=3  sample_time=0.001000
  EtherCAT Rx Var 14 : xpcethercatlib/EtherCAT PDO Receive  Priority=2  sig_name=Box 5 (ATRIAS 2.1 Leg (Medulla 1.5)).Thermistors.Thermistor 2  sig_offset=1344  sig_type=uint16  type_size=16  sig_dim=1  device_id=3  sample_time=0.001000
  EtherCAT Rx Var 15 : xpcethercatlib/EtherCAT PDO Receive  Priority=2  sig_name=Box 5 (ATRIAS 2.1 Leg (Medulla 1.5)).Thermistors.Thermistor 3  sig_offset=1360  sig_type=uint16  type_size=16  sig_dim=1  device_id=3  sample_time=0.001000
  EtherCAT Rx Var 16 : xpcethercatlib/EtherCAT PDO Receive  Priority=2  sig_name=Box 5 (ATRIAS 2.1 Leg (Medulla 1.5)).Thermistors.Thermistor 4  sig_offset=1376  sig_type=uint16  type_size=16  sig_dim=1  device_id=3  sample_time=0.001000
  EtherCAT Rx Var 17 : xpcethercatlib/EtherCAT PDO Receive  Priority=2  sig_name=Box 5 (ATRIAS 2.1 Leg (Medulla 1.5)).Thermistors.Thermistor 5  sig_offset=1392  sig_type=uint16  type_size=16  sig_dim=1  device_id=3  sample_time=0.001000
  EtherCAT Rx Var 18 : xpcethercatlib/EtherCAT PDO Receive  Priority=2  sig_name=Box 5 (ATRIAS 2.1 Leg (Medulla 1.5)).uController Status.Counter  sig_offset=1112  sig_type=uint8  type_size=8  sig_dim=1  device_id=3  sample_time=0.001000
  EtherCAT Rx Var 19 : xpcethercatlib/EtherCAT PDO Receive  Priority=2  sig_name=Box 5 (ATRIAS 2.1 Leg (Medulla 1.5)).uController Status.Error Flags  sig_offset=1120  sig_type=uint8  type_size=8  sig_dim=1  device_id=3  sample_time=0.001000
  EtherCAT Rx Var 2 : xpcethercatlib/EtherCAT PDO Receive  Priority=2  sig_name=Box 5 (ATRIAS 2.1 Leg (Medulla 1.5)).Knee Force.Knee Force 1  sig_offset=1440  sig_type=uint16  type_size=16  sig_dim=1  device_id=3  sample_time=0.001000
  EtherCAT Rx Var 20 : xpcethercatlib/EtherCAT PDO Receive  Priority=2  sig_name=Box 5 (ATRIAS 2.1 Leg (Medulla 1.5)).uController Status.ID  sig_offset=1096  sig_type=uint8  type_size=8  sig_dim=1  device_id=3  sample_time=0.001000
  EtherCAT Rx Var 21 : xpcethercatlib/EtherCAT PDO Receive  Priority=2  sig_name=Box 5 (ATRIAS 2.1 Leg (Medulla 1.5)).uController Status.Limit Switch  sig_offset=1128  sig_type=uint8  type_size=8  sig_dim=1  device_id=3  sample_time=0.001000
  EtherCAT Rx Var 22 : xpcethercatlib/EtherCAT PDO Receive  Priority=2  sig_name=Box 5 (ATRIAS 2.1 Leg (Medulla 1.5)).uController Status.State  sig_offset=1104  sig_type=uint8  type_size=8  sig_dim=1  device_id=3  sample_time=0.001000
  EtherCAT Rx Var 23 : xpcethercatlib/EtherCAT PDO Receive  Priority=2  sig_name=Box 5 (ATRIAS 2.1 Leg (Medulla 1.5)).uController Status.Toe Sensor  sig_offset=1136  sig_type=uint16  type_size=16  sig_dim=1  device_id=3  sample_time=0.001000
  EtherCAT Rx Var 3 : xpcethercatlib/EtherCAT PDO Receive  Priority=2  sig_name=Box 5 (ATRIAS 2.1 Leg (Medulla 1.5)).Knee Force.Knee Force 2  sig_offset=1456  sig_type=uint16  type_size=16  sig_dim=1  device_id=3  sample_time=0.001000
  EtherCAT Rx Var 4 : xpcethercatlib/EtherCAT PDO Receive  Priority=2  sig_name=Box 5 (ATRIAS 2.1 Leg (Medulla 1.5)).Leg Encoder.Leg Encoder  sig_offset=1200  sig_type=uint32  type_size=32  sig_dim=1  device_id=3  sample_time=0.001000
  EtherCAT Rx Var 5 : xpcethercatlib/EtherCAT PDO Receive  Priority=2  sig_name=Box 5 (ATRIAS 2.1 Leg (Medulla 1.5)).Leg Encoder.Leg Encoder Timestamp  sig_offset=1232  sig_type=uint16  type_size=16  sig_dim=1  device_id=3  sample_time=0.001000
  EtherCAT Rx Var 6 : xpcethercatlib/EtherCAT PDO Receive  Priority=2  sig_name=Box 5 (ATRIAS 2.1 Leg (Medulla 1.5)).Measured Current.Amp 1 Measured Current  sig_offset=1408  sig_type=int16  type_size=16  sig_dim=1  device_id=3  sample_time=0.001000
  EtherCAT Rx Var 7 : xpcethercatlib/EtherCAT PDO Receive  Priority=2  sig_name=Box 5 (ATRIAS 2.1 Leg (Medulla 1.5)).Measured Current.Amp 2 Measured Current  sig_offset=1424  sig_type=int16  type_size=16  sig_dim=1  device_id=3  sample_time=0.001000
  EtherCAT Rx Var 8 : xpcethercatlib/EtherCAT PDO Receive  Priority=2  sig_name=Box 5 (ATRIAS 2.1 Leg (Medulla 1.5)).Motor Encoder.Motor Encoder  sig_offset=1152  sig_type=uint32  type_size=32  sig_dim=1  device_id=3  sample_time=0.001000
  EtherCAT Rx Var 9 : xpcethercatlib/EtherCAT PDO Receive  Priority=2  sig_name=Box 5 (ATRIAS 2.1 Leg (Medulla 1.5)).Motor Encoder.Motor Encoder Timestamp  sig_offset=1184  sig_type=uint16  type_size=16  sig_dim=1  device_id=3  sample_time=0.001000
  EtherCAT Tx Var 3 : xpcethercatlib/EtherCAT PDO Transmit   Priority=3  sig_name=Box 5 (ATRIAS 2.1 Leg (Medulla 1.5)).uControllerInput.Command  sig_offset=1096  sig_type=uint8  type_size=8  sig_dim=1  device_id=3  sample_time=0.001000
  EtherCAT Tx Var 4 : xpcethercatlib/EtherCAT PDO Transmit   Priority=3  sig_name=Box 5 (ATRIAS 2.1 Leg (Medulla 1.5)).uControllerInput.Counter  sig_offset=1104  sig_type=uint16  type_size=16  sig_dim=1  device_id=3  sample_time=0.001000
  EtherCAT Tx Var 5 : xpcethercatlib/EtherCAT PDO Transmit   Priority=3  sig_name=Box 5 (ATRIAS 2.1 Leg (Medulla 1.5)).uControllerInput.Motor Current  sig_offset=1120  sig_type=int32  type_size=32  sig_dim=1  device_id=3  sample_time=0.001000
  Mux1 : Mux  Inputs=2
  Mux2 : Mux  Inputs=2
  Mux5 : Mux  Inputs=6
  LegEncoder : Outport
  MotorEncoder : Outport  Port=2
  ToeSensor : Outport  Port=3
  LimitSwitch : Outport  Port=4
  ID : Outport  Port=5
  State : Outport  Port=6
  Counter : Outport  Port=7
  ErrorFlags : Outport  Port=8
  IncEncoder : Outport  Port=9
  LegEncoderTimestamp : Outport  Port=10
  MotorEncoderTimestamp : Outport  Port=11
  IncEncoderTimestamp : Outport  Port=12
  MotorVoltage : Outport  Port=13
  LogicVoltage : Outport  Port=14
  Thermistors : Outport  Port=15
  AmpMeasuredCurrent : Outport  Port=16
  KneeForce : Outport  Port=17
  wires:
  Mux2/1 -> KneeForce/1
  EtherCAT Rx Var 3/1 -> Mux2/2
  EtherCAT Rx Var 7/1 -> Mux1/2
  Mux1/1 -> AmpMeasuredCurrent/1
  Mux5/1 -> Thermistors/1
  EtherCAT Rx Var 12/1 -> Mux5/1
  MotorCmd/1 -> Data Type Conversion5/1
  MedullaCounter/1 -> Data Type Conversion4/1
  MedullaCmd/1 -> Data Type Conversion3/1
  EtherCAT Rx Var 23/1 -> ToeSensor/1
  EtherCAT Rx Var 22/1 -> State/1
  EtherCAT Rx Var 21/1 -> LimitSwitch/1
  EtherCAT Rx Var 20/1 -> ID/1
  EtherCAT Rx Var 19/1 -> ErrorFlags/1
  EtherCAT Rx Var 18/1 -> Counter/1
  EtherCAT Rx Var 17/1 -> Mux5/6
  EtherCAT Rx Var 16/1 -> Mux5/5
  EtherCAT Rx Var 15/1 -> Mux5/4
  EtherCAT Rx Var 14/1 -> Mux5/3
  EtherCAT Rx Var 13/1 -> Mux5/2
  EtherCAT Rx Var 11/1 -> MotorVoltage/1
  EtherCAT Rx Var 10/1 -> LogicVoltage/1
  EtherCAT Rx Var 9/1 -> MotorEncoderTimestamp/1
  EtherCAT Rx Var 8/1 -> MotorEncoder/1
  EtherCAT Rx Var 6/1 -> Mux1/1
  EtherCAT Rx Var 5/1 -> LegEncoderTimestamp/1
  EtherCAT Rx Var 4/1 -> LegEncoder/1
  EtherCAT Rx Var 2/1 -> Mux2/1
  EtherCAT Rx Var 1/1 -> IncEncoderTimestamp/1
  "EtherCAT Rx Var "/1 -> IncEncoder/1
  Data Type Conversion5/1 -> EtherCAT Tx Var 5/1
  Data Type Conversion4/1 -> EtherCAT Tx Var 4/1
  Data Type Conversion3/1 -> EtherCAT Tx Var 3/1

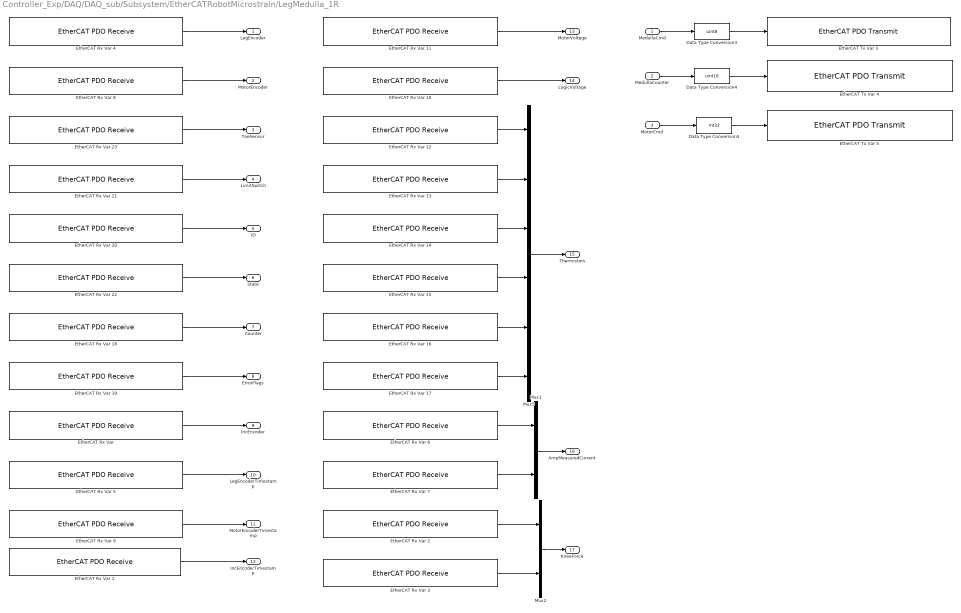
== system Controller_Exp/DAQ/DAQ_sub/Subsystem/EtherCATRobotMicrostrain/LegMedulla_1R ==
  MedullaCmd : Inport
  MedullaCounter : Inport  Port=2
  MotorCmd : Inport  Port=3
  Data Type Conversion3 : DataTypeConversion  OutDataTypeStr=uint8  RndMeth=Simplest
  Data Type Conversion4 : DataTypeConversion  OutDataTypeStr=uint16  RndMeth=Simplest
  Data Type Conversion5 : DataTypeConversion  OutDataTypeStr=int32  RndMeth=Simplest
  "EtherCAT Rx Var " : xpcethercatlib/EtherCAT PDO Receive  Priority=2  sig_name=Box 8 (ATRIAS 2.1 Leg (Medulla 1.5)).Incremental Encoder.Incremental Encoder  sig_offset=2376  sig_type=uint16  type_size=16  sig_dim=1  device_id=3  sample_time=0.001000
  EtherCAT Rx Var 1 : xpcethercatlib/EtherCAT PDO Receive  Priority=2  sig_name=Box 8 (ATRIAS 2.1 Leg (Medulla 1.5)).Incremental Encoder.Incremental Encoder Timestamp  sig_offset=2392  sig_type=uint16  type_size=16  sig_dim=1  device_id=3  sample_time=0.001000
  EtherCAT Rx Var 10 : xpcethercatlib/EtherCAT PDO Receive  Priority=2  sig_name=Box 8 (ATRIAS 2.1 Leg (Medulla 1.5)).Power.Logic Voltage  sig_offset=2424  sig_type=uint16  type_size=16  sig_dim=1  device_id=3  sample_time=0.001000
  EtherCAT Rx Var 11 : xpcethercatlib/EtherCAT PDO Receive  Priority=2  sig_name=Box 8 (ATRIAS 2.1 Leg (Medulla 1.5)).Power.Motor Voltage  sig_offset=2408  sig_type=uint16  type_size=16  sig_dim=1  device_id=3  sample_time=0.001000
  EtherCAT Rx Var 12 : xpcethercatlib/EtherCAT PDO Receive  Priority=2  sig_name=Box 8 (ATRIAS 2.1 Leg (Medulla 1.5)).Thermistors.Thermistor 0  sig_offset=2440  sig_type=uint16  type_size=16  sig_dim=1  device_id=3  sample_time=0.001000
  EtherCAT Rx Var 13 : xpcethercatlib/EtherCAT PDO Receive  Priority=2  sig_name=Box 8 (ATRIAS 2.1 Leg (Medulla 1.5)).Thermistors.Thermistor 1  sig_offset=2456  sig_type=uint16  type_size=16  sig_dim=1  device_id=3  sample_time=0.001000
  EtherCAT Rx Var 14 : xpcethercatlib/EtherCAT PDO Receive  Priority=2  sig_name=Box 8 (ATRIAS 2.1 Leg (Medulla 1.5)).Thermistors.Thermistor 2  sig_offset=2472  sig_type=uint16  type_size=16  sig_dim=1  device_id=3  sample_time=0.001000
  EtherCAT Rx Var 15 : xpcethercatlib/EtherCAT PDO Receive  Priority=2  sig_name=Box 8 (ATRIAS 2.1 Leg (Medulla 1.5)).Thermistors.Thermistor 3  sig_offset=2488  sig_type=uint16  type_size=16  sig_dim=1  device_id=3  sample_time=0.001000
  EtherCAT Rx Var 16 : xpcethercatlib/EtherCAT PDO Receive  Priority=2  sig_name=Box 8 (ATRIAS 2.1 Leg (Medulla 1.5)).Thermistors.Thermistor 4  sig_offset=2504  sig_type=uint16  type_size=16  sig_dim=1  device_id=3  sample_time=0.001000
  EtherCAT Rx Var 17 : xpcethercatlib/EtherCAT PDO Receive  Priority=2  sig_name=Box 8 (ATRIAS 2.1 Leg (Medulla 1.5)).Thermistors.Thermistor 5  sig_offset=2520  sig_type=uint16  type_size=16  sig_dim=1  device_id=3  sample_time=0.001000
  EtherCAT Rx Var 18 : xpcethercatlib/EtherCAT PDO Receive  Priority=2  sig_name=Box 8 (ATRIAS 2.1 Leg (Medulla 1.5)).uController Status.Counter  sig_offset=2240  sig_type=uint8  type_size=8  sig_dim=1  device_id=3  sample_time=0.001000
  EtherCAT Rx Var 19 : xpcethercatlib/EtherCAT PDO Receive  Priority=2  sig_name=Box 8 (ATRIAS 2.1 Leg (Medulla 1.5)).uController Status.Error Flags  sig_offset=2248  sig_type=uint8  type_size=8  sig_dim=1  device_id=3  sample_time=0.001000
  EtherCAT Rx Var 2 : xpcethercatlib/EtherCAT PDO Receive  Priority=2  sig_name=Box 8 (ATRIAS 2.1 Leg (Medulla 1.5)).Knee Force.Knee Force 1  sig_offset=2568  sig_type=uint16  type_size=16  sig_dim=1  device_id=3  sample_time=0.001000
  EtherCAT Rx Var 20 : xpcethercatlib/EtherCAT PDO Receive  Priority=2  sig_name=Box 8 (ATRIAS 2.1 Leg (Medulla 1.5)).uController Status.State  sig_offset=2232  sig_type=uint8  type_size=8  sig_dim=1  device_id=3  sample_time=0.001000
  EtherCAT Rx Var 21 : xpcethercatlib/EtherCAT PDO Receive  Priority=2  sig_name=Box 8 (ATRIAS 2.1 Leg (Medulla 1.5)).uController Status.Limit Switch  sig_offset=2256  sig_type=uint8  type_size=8  sig_dim=1  device_id=3  sample_time=0.001000
  EtherCAT Rx Var 22 : xpcethercatlib/EtherCAT PDO Receive  Priority=2  sig_name=Box 8 (ATRIAS 2.1 Leg (Medulla 1.5)).uController Status.State  sig_offset=2232  sig_type=uint8  type_size=8  sig_dim=1  device_id=3  sample_time=0.001000
  EtherCAT Rx Var 23 : xpcethercatlib/EtherCAT PDO Receive  Priority=2  sig_name=Box 8 (ATRIAS 2.1 Leg (Medulla 1.5)).uController Status.Toe Sensor  sig_offset=2264  sig_type=uint16  type_size=16  sig_dim=1  device_id=3  sample_time=0.001000
  EtherCAT Rx Var 3 : xpcethercatlib/EtherCAT PDO Receive  Priority=2  sig_name=Box 8 (ATRIAS 2.1 Leg (Medulla 1.5)).Knee Force.Knee Force 2  sig_offset=2584  sig_type=uint16  type_size=16  sig_dim=1  device_id=3  sample_time=0.001000
  EtherCAT Rx Var 4 : xpcethercatlib/EtherCAT PDO Receive  Priority=2  sig_name=Box 8 (ATRIAS 2.1 Leg (Medulla 1.5)).Leg Encoder.Leg Encoder  sig_offset=2328  sig_type=uint32  type_size=32  sig_dim=1  device_id=3  sample_time=0.001000
  EtherCAT Rx Var 5 : xpcethercatlib/EtherCAT PDO Receive  Priority=2  sig_name=Box 8 (ATRIAS 2.1 Leg (Medulla 1.5)).Leg Encoder.Leg Encoder Timestamp  sig_offset=2360  sig_type=uint16  type_size=16  sig_dim=1  device_id=3  sample_time=0.001000
  EtherCAT Rx Var 6 : xpcethercatlib/EtherCAT PDO Receive  Priority=2  sig_name=Box 8 (ATRIAS 2.1 Leg (Medulla 1.5)).Measured Current.Amp 1 Measured Current  sig_offset=2536  sig_type=int16  type_size=16  sig_dim=1  device_id=3  sample_time=0.001000
  EtherCAT Rx Var 7 : xpcethercatlib/EtherCAT PDO Receive  Priority=2  sig_name=Box 8 (ATRIAS 2.1 Leg (Medulla 1.5)).Measured Current.Amp 2 Measured Current  sig_offset=2552  sig_type=int16  type_size=16  sig_dim=1  device_id=3  sample_time=0.001000
  EtherCAT Rx Var 8 : xpcethercatlib/EtherCAT PDO Receive  Priority=2  sig_name=Box 8 (ATRIAS 2.1 Leg (Medulla 1.5)).Motor Encoder.Motor Encoder  sig_offset=2280  sig_type=uint32  type_size=32  sig_dim=1  device_id=3  sample_time=0.001000
  EtherCAT Rx Var 9 : xpcethercatlib/EtherCAT PDO Receive  Priority=2  sig_name=Box 8 (ATRIAS 2.1 Leg (Medulla 1.5)).Motor Encoder.Motor Encoder Timestamp  sig_offset=2312  sig_type=uint16  type_size=16  sig_dim=1  device_id=3  sample_time=0.001000
  EtherCAT Tx Var 3 : xpcethercatlib/EtherCAT PDO Transmit   Priority=3  sig_name=Box 8 (ATRIAS 2.1 Leg (Medulla 1.5)).uControllerInput.Command  sig_offset=2224  sig_type=uint8  type_size=8  sig_dim=1  device_id=3  sample_time=0.001000
  EtherCAT Tx Var 4 : xpcethercatlib/EtherCAT PDO Transmit   Priority=3  sig_name=Box 8 (ATRIAS 2.1 Leg (Medulla 1.5)).uControllerInput.Counter  sig_offset=2232  sig_type=uint16  type_size=16  sig_dim=1  device_id=3  sample_time=0.001000
  EtherCAT Tx Var 5 : xpcethercatlib/EtherCAT PDO Transmit   Priority=3  sig_name=Box 8 (ATRIAS 2.1 Leg (Medulla 1.5)).uControllerInput.Motor Current  sig_offset=2248  sig_type=int32  type_size=32  sig_dim=1  device_id=3  sample_time=0.001000
  Mux1 : Mux  Inputs=2
  Mux2 : Mux  Inputs=2
  Mux5 : Mux  Inputs=6
  LegEncoder : Outport
  MotorEncoder : Outport  Port=2
  ToeSensor : Outport  Port=3
  LimitSwitch : Outport  Port=4
  ID : Outport  Port=5
  State : Outport  Port=6
  Counter : Outport  Port=7
  ErrorFlags : Outport  Port=8
  IncEncoder : Outport  Port=9
  LegEncoderTimestamp : Outport  Port=10
  MotorEncoderTimestamp : Outport  Port=11
  IncEncoderTimestamp : Outport  Port=12
  MotorVoltage : Outport  Port=13
  LogicVoltage : Outport  Port=14
  Thermistors : Outport  Port=15
  AmpMeasuredCurrent : Outport  Port=16
  KneeForce : Outport  Port=17
  wires:
  Mux2/1 -> KneeForce/1
  Mux1/1 -> AmpMeasuredCurrent/1
  Mux5/1 -> Thermistors/1
  MotorCmd/1 -> Data Type Conversion5/1
  MedullaCounter/1 -> Data Type Conversion4/1
  MedullaCmd/1 -> Data Type Conversion3/1
  EtherCAT Rx Var 23/1 -> ToeSensor/1
  EtherCAT Rx Var 22/1 -> State/1
  EtherCAT Rx Var 21/1 -> LimitSwitch/1
  EtherCAT Rx Var 20/1 -> ID/1
  EtherCAT Rx Var 19/1 -> ErrorFlags/1
  EtherCAT Rx Var 18/1 -> Counter/1
  EtherCAT Rx Var 17/1 -> Mux5/6
  EtherCAT Rx Var 16/1 -> Mux5/5
  EtherCAT Rx Var 15/1 -> Mux5/4
  EtherCAT Rx Var 14/1 -> Mux5/3
  EtherCAT Rx Var 13/1 -> Mux5/2
  EtherCAT Rx Var 12/1 -> Mux5/1
  EtherCAT Rx Var 11/1 -> MotorVoltage/1
  EtherCAT Rx Var 10/1 -> LogicVoltage/1
  EtherCAT Rx Var 9/1 -> MotorEncoderTimestamp/1
  EtherCAT Rx Var 8/1 -> MotorEncoder/1
  EtherCAT Rx Var 7/1 -> Mux1/2
  EtherCAT Rx Var 6/1 -> Mux1/1
  EtherCAT Rx Var 5/1 -> LegEncoderTimestamp/1
  EtherCAT Rx Var 4/1 -> LegEncoder/1
  EtherCAT Rx Var 3/1 -> Mux2/2
  EtherCAT Rx Var 2/1 -> Mux2/1
  EtherCAT Rx Var 1/1 -> IncEncoderTimestamp/1
  "EtherCAT Rx Var "/1 -> IncEncoder/1
  Data Type Conversion5/1 -> EtherCAT Tx Var 5/1
  Data Type Conversion4/1 -> EtherCAT Tx Var 4/1
  Data Type Conversion3/1 -> EtherCAT Tx Var 3/1
